simulink model "sf_tictacflow_sim"  (Simulink 6.0)
settings: Solver=ode45  StartTime=0.0  StopTime=inf  RelTol=1e-3
libraries: simulink3 x1
settings Model: CovMetricSettings=dcmtr  Creator=The MathWorks Inc.  LastModifiedBy=batserve  ExtModeTrigMode=oneshot  ExtModeArmWhenConnect=off  ExtModeAutoUpdateStatusClock=off
settings DataIOCC: LimitDataPoints=off  SaveOutput=off  SaveTime=off
settings OptimizationCC: BlockReduction=off  BooleanDataType=off
settings DebuggingCC: CheckExecutionContextPreStartOutputMsg=on  CheckExecutionContextRuntimeOutputMsg=on  SolverPrmCheckMsg=none
settings HardwareCC: TargetUnknown=on

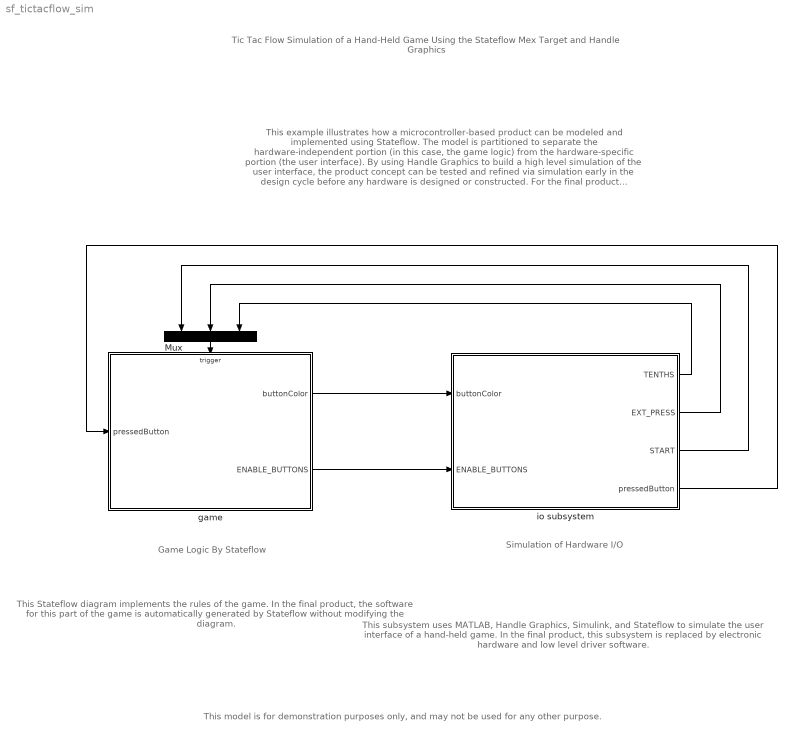
== system sf_tictacflow_sim ==
  note: Tic Tac Flow
      | Simulation of a Hand-Held Game
      | Using the Stateflow Mex Target
      | and Handle Graphics
  note: This model is for demonstration purposes only, and may not be used for any other purpose.
  note: This Stateflow diagram implements
      | the rules of the game.
      |
      | In the final product, the software for this
      | part of the game is automatically generated
      |  by Stateflow without modifying the diagram.
  note: Game Logic By Stateflow
  note: This subsystem uses MATLAB, Handle
      | Graphics, Simulink, and Stateflow
      |  to simulate the user interface of a
      | hand-held game.
      |
      | In the final product, this subsystem is
      | replaced by electronic hardware and
      | low level driver software.
  note: Simulation of Hardware I/O
  note: This example illustrates how a microcontroller-based product can be modeled and implemented using Stateflow.
      |
      | The model is partitioned to separate the hardware-independent portion (in
      | this case, the game logic) from the hardware-specific portion (the user interface).
      | By using Handle Graphics to build a high level simulation of the user interface, the product concept can
      |  be tested and refined via simulation early in the design cycle before any hardware is designed or constructed.
      | For the final product implementation, the hardware-independent portion is implemented automatically
      |  by Stateflow, while the hardware-specific portion is replaced by actual hardware and low-level driver software.
  Mux : Mux  Orientation=down  Inputs=3
  game : Stateflow chart  TreatAsAtomicUnit=on  PropExecContextAcrossSSBoundary=on
  io subsystem : Subsystem  StopFcn=if ishandle(1.000000); delete(1.000000); end;  PropExecContextAcrossSSBoundary=on
  wires:
  io subsystem/4(pressedButton) -> game/1(pressedButton)
  io subsystem/3(START) -> Mux/1
  io subsystem/2(EXT_PRESS) -> Mux/2
  game/2(ENABLE_BUTTONS) -> io subsystem/2(ENABLE_BUTTONS)
  Mux/1 -> game/Trigger
  game/1(buttonColor) -> io subsystem/1(buttonColor)
  io subsystem/1(TENTHS) -> Mux/3

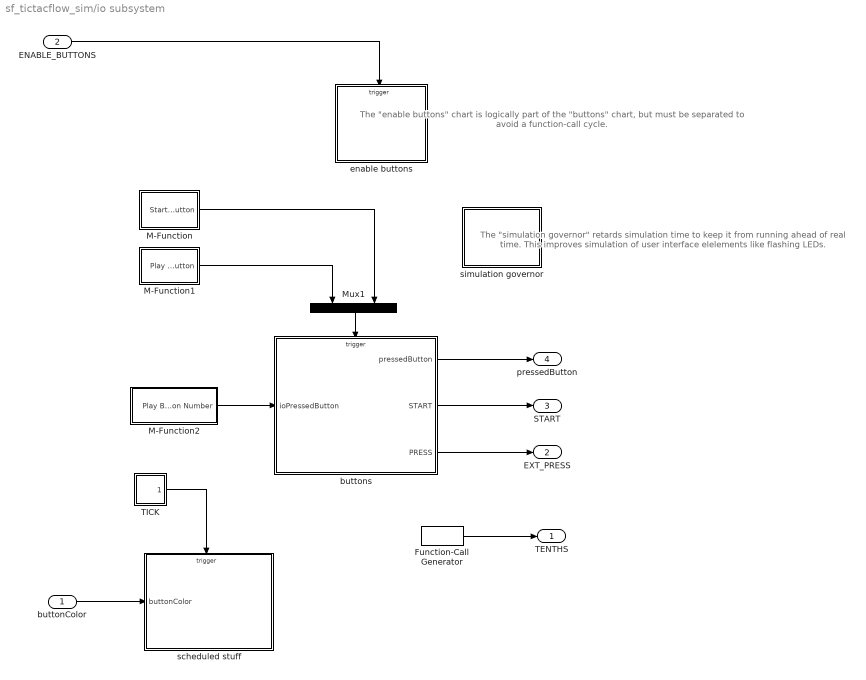
== system sf_tictacflow_sim/io subsystem ==
  note: The "enable buttons" chart is logically part of the
      | "buttons" chart, but must be separated to avoid
      | a function-call cycle.
  note: The "simulation governor" retards simulation time
      | to keep it from running ahead of real time.  This
      | improves simulation of user interface elelements
      | like flashing LEDs.
  buttonColor : Inport  Port=1  LatchInput=off
  ENABLE_BUTTONS : Inport  Port=2  LatchInput=off
  Function-Call Generator : simulink3/Signals & Systems/Function-Call Generator  sample_time=0.1  numberOfIterations=1
  M-Function : Subsystem  PropExecContextAcrossSSBoundary=on
  M-Function1 : Subsystem  PropExecContextAcrossSSBoundary=on
  M-Function2 : Subsystem  PropExecContextAcrossSSBoundary=on
  Mux1 : Mux  Orientation=down  Inputs=2
  TICK : Subsystem  PropExecContextAcrossSSBoundary=on  mask(Pulse Generator){period=1/20, duty=50, amplitude=1, start=0}
      mask prompts: period "Period (secs):"; duty "Duty cycle (% of period):"; start "Start time:"
      mask help: Pulse Generator
      mask Help: Pulse generator which ensures pulse transitions are hit. Provides a vector of pulses when the height is entered as a vector.  Unmask to see how it works.
      mask Display: plot(0,0,100,100,[95,90,90,75,75,60,60,45,45,30,30,15,15,5],[25,25,75,75,25,25,75,75,25,25,75,75,25,25]);
  buttons : Stateflow chart  TreatAsAtomicUnit=on  PropExecContextAcrossSSBoundary=on
  enable buttons : Stateflow chart  TreatAsAtomicUnit=on  PropExecContextAcrossSSBoundary=on
  scheduled stuff : Stateflow chart  TreatAsAtomicUnit=on  PropExecContextAcrossSSBoundary=on
  simulation governor : Subsystem  PropExecContextAcrossSSBoundary=on
  TENTHS : Outport
  EXT_PRESS : Outport  Port=2
  START : Outport  Port=3
  pressedButton : Outport  Port=4
  wires:
  buttons/3(PRESS) -> EXT_PRESS/1
  Mux1/1 -> buttons/Trigger
  buttons/1(pressedButton) -> pressedButton/1
  buttons/2(START) -> START/1
  Function-Call Generator/1 -> TENTHS/1
  M-Function2/1(Play Button Number) -> buttons/1(ioPressedButton)
  buttonColor/1 -> scheduled stuff/1(buttonColor)
  TICK/1(Out1) -> scheduled stuff/Trigger
  M-Function/1(Start Button) -> Mux1/2
  M-Function1/1(Play Button) -> Mux1/1
  ENABLE_BUTTONS/1 -> enable buttons/Trigger

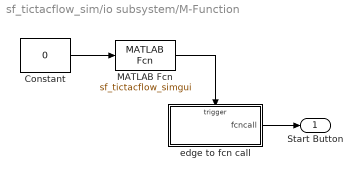
== system sf_tictacflow_sim/io subsystem/M-Function ==
  Constant : Constant  Value=0
  MATLAB Fcn : MATLABFcn  MATLABFcn=sf_tictacflow_simgui
  edge to fcn call : Stateflow chart  TreatAsAtomicUnit=on  PropExecContextAcrossSSBoundary=on
  Start Button : Outport
  wires:
  Constant/1 -> MATLAB Fcn/1
  MATLAB Fcn/1 -> edge to fcn call/Trigger
  edge to fcn call/1(fcncall) -> Start Button/1

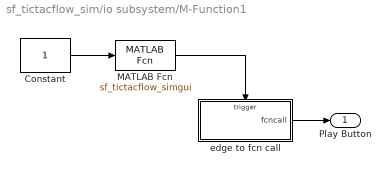
== system sf_tictacflow_sim/io subsystem/M-Function1 ==
  Constant : Constant
  MATLAB Fcn : MATLABFcn  MATLABFcn=sf_tictacflow_simgui
  edge to fcn call : Stateflow chart  TreatAsAtomicUnit=on  PropExecContextAcrossSSBoundary=on
  Play Button : Outport
  wires:
  Constant/1 -> MATLAB Fcn/1
  MATLAB Fcn/1 -> edge to fcn call/Trigger
  edge to fcn call/1(fcncall) -> Play Button/1

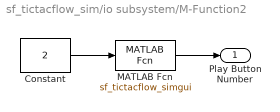
== system sf_tictacflow_sim/io subsystem/M-Function2 ==
  Constant : Constant  Value=2
  MATLAB Fcn : MATLABFcn  MATLABFcn=sf_tictacflow_simgui
  Play Button Number : Outport
  wires:
  MATLAB Fcn/1 -> Play Button Number/1
  Constant/1 -> MATLAB Fcn/1

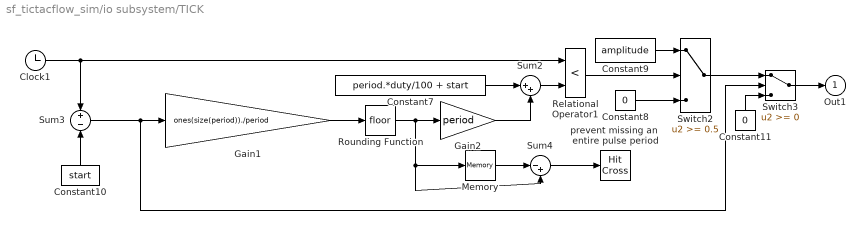
== system sf_tictacflow_sim/io subsystem/TICK ==
  Clock1 : Clock
      settings: Decimation=10
  Constant10 : Constant  Orientation=up  Value=start
  Constant11 : Constant  Orientation=up  Value=0
  Constant7 : Constant  Value=period.*duty/100 + start
  Constant8 : Constant  Value=0
  Constant9 : Constant  Value=amplitude
  Gain1 : Gain  Gain=ones(size(period))./period  SaturateOnIntegerOverflow=on
  Gain2 : Gain  Gain=period  SaturateOnIntegerOverflow=on
  Memory : Memory
  Relational Operator1 : RelationalOperator  Operator=<  InputSameDT=on
  Rounding Function : Rounding
  Sum2 : Sum  Inputs=|++  SaturateOnIntegerOverflow=on  InputSameDT=on
  Sum3 : Sum  Inputs=+-  SaturateOnIntegerOverflow=on  InputSameDT=on
  Sum4 : Sum  Inputs=|-+  SaturateOnIntegerOverflow=on  InputSameDT=on
  Switch2 : Switch  Threshold=0.5  SaturateOnIntegerOverflow=on  InputSameDT=on
  Switch3 : Switch  SaturateOnIntegerOverflow=on  InputSameDT=on
  prevent missing an  entire pulse period : HitCross  HitCrossingOffset=1  ShowOutputPort=off
  Out1 : Outport
  wires:
  Constant10/1 -> Sum3/2
  Sum3/1 -> Gain1/1, Switch3/2
  Clock1/1 -> Relational Operator1/1, Sum3/1
  Sum2/1 -> Relational Operator1/2
  Gain1/1 -> Rounding Function/1
  Constant7/1 -> Sum2/1
  Gain2/1 -> Sum2/2
  Rounding Function/1 -> Sum4/2, Memory/1, Gain2/1
  Switch3/1 -> Out1/1
  Relational Operator1/1 -> Switch2/2
  Constant8/1 -> Switch2/3
  Constant9/1 -> Switch2/1
  Constant11/1 -> Switch3/3
  Switch2/1 -> Switch3/1
  Sum4/1 -> prevent missing an  entire pulse period/1
  Memory/1 -> Sum4/1

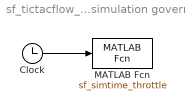
== system sf_tictacflow_sim/io subsystem/simulation governor ==
  Clock : Clock
      settings: Decimation=10
  MATLAB Fcn : MATLABFcn  MATLABFcn=sf_simtime_throttle  OutputDimensions=0
  wires:
  Clock/1 -> MATLAB Fcn/1

== stateflow chart io subsystem/M-Function1/edge to fcn call ==
  (default) -> (junction 3) : { fcncall; }
  events: edge input EITHER_EDGE_EVENT; fcncall output FUNCTION_CALL_EVENT

== stateflow chart io subsystem/M-Function/edge to fcn call ==
  (default) -> (junction 9) : { fcncall; }
  events: edge input EITHER_EDGE_EVENT; fcncall output FUNCTION_CALL_EVENT

== stateflow chart io subsystem/enable buttons ==
  settings: executeAtInitialization=1
  state enable_buttons
    on ENABLE_BUTTONS:
    ml.set(buttonH[0],'Enable','On');
    ml.set(buttonH[1],'Enable','On');
    ml.set(buttonH[2],'Enable','On');
    ml.set(buttonH[3],'Enable','On');
    ml.set(buttonH[4],'Enable','On');
    ml.set(buttonH[5],'Enable','On');
    ml.set(buttonH[6],'Enable','On');
    ml.set(buttonH[7],'Enable','On');
    ml.set(buttonH[8],'Enable','On');
  events: ENABLE_BUTTONS input FUNCTION_CALL_EVENT

== stateflow chart game ==
  settings: executeAtInitialization=1
  state button_7 [parallel]
    state enabled
      buttonColor[thisButton] = DARK;
    state disabled
    state active
      state red
        buttonColor[thisButton] = RED;
        TURN;
      state green
        buttonColor[thisButton] = GREEN;
        TURN;
      (junction 85) -> button_7.active.red
      (junction 85) -> button_7.active.green : [in(turn.green)]
    button_7 -> button_7.disabled : GAME_OVER
    button_7 -> button_7.enabled : START
    (default) -> button_7.enabled
    button_7.active -> button_7.enabled : at(7,TURN)
    button_7.enabled -> (junction 85) : PRESS
  state button_0 [parallel]
    state disabled
    state enabled
      buttonColor[thisButton] = DARK;
    state active
      state red
        buttonColor[thisButton] = RED;
        TURN;
      state green
        buttonColor[thisButton] = GREEN;
        TURN;
      (junction 86) -> button_0.active.red
      (junction 86) -> button_0.active.green : [in(turn.green)]
    button_0 -> button_0.disabled : GAME_OVER
    button_0 -> button_0.enabled : START
    (default) -> button_0.enabled
    button_0.active -> button_0.enabled : at(7,TURN)
    button_0.enabled -> (junction 86) : PRESS
  state button_5 [parallel]
    state disabled
    state enabled
      buttonColor[thisButton] = DARK;
    state active
      state red
        buttonColor[thisButton] = RED;
        TURN;
      state green
        buttonColor[thisButton] = GREEN;
        TURN;
      (junction 87) -> button_5.active.red
      (junction 87) -> button_5.active.green : [in(turn.green)]
    button_5 -> button_5.enabled : START
    button_5 -> button_5.disabled : GAME_OVER
    (default) -> button_5.enabled
    button_5.active -> button_5.enabled : at(7,TURN)
    button_5.enabled -> (junction 87) : PRESS
  state button_2 [parallel]
    state disabled
    state enabled
      buttonColor[thisButton] = DARK;
    state active
      state red
        buttonColor[thisButton] = RED;
        TURN;
      state green
        buttonColor[thisButton] = GREEN;
        TURN;
      (junction 88) -> button_2.active.red
      (junction 88) -> button_2.active.green : [in(turn.green)]
    button_2 -> button_2.disabled : GAME_OVER
    button_2 -> button_2.enabled : START
    (default) -> button_2.enabled
    button_2.active -> button_2.enabled : at(7,TURN)
    button_2.enabled -> (junction 88) : PRESS
  state button_4 [parallel]
    state disabled
    state enabled
      buttonColor[thisButton] = DARK;
    state active
      state red
        buttonColor[thisButton] = RED;
        TURN;
      state green
        buttonColor[thisButton] = GREEN;
        TURN;
      (junction 89) -> button_4.active.red
      (junction 89) -> button_4.active.green : [in(turn.green)]
    button_4 -> button_4.enabled : START
    button_4 -> button_4.disabled : GAME_OVER
    (default) -> button_4.enabled
    button_4.active -> button_4.enabled : at(7,TURN)
    button_4.enabled -> (junction 89) : PRESS
  state button_6 [parallel]
    state disabled
    state enabled
      buttonColor[thisButton] = DARK;
    state active
      state red
        buttonColor[thisButton] = RED;
        TURN;
      state green
        buttonColor[thisButton] = GREEN;
        TURN;
      (junction 90) -> button_6.active.red
      (junction 90) -> button_6.active.green : [in(turn.green)]
    button_6 -> button_6.enabled : START
    button_6 -> button_6.disabled : GAME_OVER
    (default) -> button_6.enabled
    button_6.active -> button_6.enabled : at(7,TURN)
    button_6.enabled -> (junction 90) : PRESS
  state button_3 [parallel]
    state disabled
    state enabled
      buttonColor[thisButton] = DARK;
    state active
      state red
        buttonColor[thisButton] = RED;
        TURN;
      state green
        buttonColor[thisButton] = GREEN;
        TURN;
      (junction 91) -> button_3.active.red
      (junction 91) -> button_3.active.green : [in(turn.green)]
    button_3 -> button_3.enabled : START
    button_3 -> button_3.disabled : GAME_OVER
    (default) -> button_3.enabled
    button_3.active -> button_3.enabled : at(7,TURN)
    button_3.enabled -> (junction 91) : PRESS
  state button_8 [parallel]
    state disabled
    state enabled
      buttonColor[thisButton] = DARK;
    state active
      state red
        buttonColor[thisButton] = RED;
        TURN;
      state green
        buttonColor[thisButton] = GREEN;
        TURN;
      (junction 92) -> button_8.active.red
      (junction 92) -> button_8.active.green : [in(turn.green)]
    button_8 -> button_8.enabled : START
    button_8 -> button_8.disabled : GAME_OVER
    (default) -> button_8.enabled
    button_8.active -> button_8.enabled : at(7,TURN)
    button_8.enabled -> (junction 92) : PRESS
  state button_1 [parallel]
    state disabled
    state enabled
      buttonColor[thisButton] = DARK;
    state active
      state red
        buttonColor[thisButton] = RED;
        TURN;
      state green
        buttonColor[thisButton] = GREEN;
        TURN;
      (junction 93) -> button_1.active.red
      (junction 93) -> button_1.active.green : [in(turn.green)]
    button_1 -> button_1.enabled : START
    button_1 -> button_1.disabled : GAME_OVER
    (default) -> button_1.enabled
    button_1.active -> button_1.enabled : at(7,TURN)
    button_1.enabled -> (junction 93) : PRESS
  state turn [parallel]
    state red
      buttonColor[9] = RED;
      on every(2,TENTHS):
      buttonColor[9] ^= RED;
    state move = choose_move() [function]
      (default) -> (junction 94) : /* try to win on this move */
          | { move = 12 - gameState[1] - gameState[3]; }
      (junction 94) -> (junction 95) : [ make_move_if_available(move) ]
      (junction 94) -> (junction 96) : /* else try to block opponent from winning next move */
          | { move = 12 - gameState[0] - gameState[2]; }
      (junction 96) -> (junction 97) : [ make_move_if_available(move) ]
      (junction 96) -> (junction 98) : /* else make a random  move */
          | { move = seed; }
      (junction 99) -> (junction 98)
      (junction 98) -> (junction 100) : {
          |   /* simple linear congruential
          |      pseudo-random sequence:
          |      x = (5x + 3) mod 16 */
          |   move += move << 2;
          |   move += 3;
          |   move &= 0xf;
          | }
      (junction 101) -> (junction 99)
      (junction 100) -> (junction 101) : [!make_move_if_available(move)]
      (junction 100) -> (junction 102) : { seed = move; }
    state game_over
      GAME_OVER;
      state on
        buttonColor[gameState[0]] = winColor;
        buttonColor[gameState[2]] = winColor;
        buttonColor[gameState[4]] = winColor;
      state off
        buttonColor[gameState[0]] = 0;
        buttonColor[gameState[2]] = 0;
        buttonColor[gameState[4]] = 0;
      (default) -> on : { winColor = buttonColor[gameState[0]]; }
      off -> on : after(1,TENTHS)
      on -> off : after(3,TENTHS)
    state yes = is_a_winner() [function]
      (default) -> (junction 103) : { yes =((gameState[0] + gameState[2] + gameState[4]) == 12); }
    state shift_game_state(magicNumber) [function]
      (default) -> (junction 104) : {
          |   gameState[5] = gameState[4];
          |   gameState[4] = gameState[3];
          |   gameState[3] = gameState[2];
          |   gameState[2] = gameState[1];
          |   gameState[1] = gameState[0];
          |   gameState[0] = magicNumber;
          | }
    state yes = make_move_if_available(move) [function]
      (default) -> (junction 105)
      (junction 105) -> (junction 106) : [ move == 0 && in(button_0.enabled)] { shift_game_state(move); send(PRESS,button_0);}
      (junction 105) -> (junction 107)
      (junction 106) -> (junction 108)
      (junction 107) -> (junction 108) : [ move == 1 && in(button_1.enabled)] { shift_game_state(move); send(PRESS,button_1);}
      (junction 107) -> (junction 109)
      (junction 108) -> (junction 110)
      (junction 109) -> (junction 110) : [ move == 2 && in(button_2.enabled)] { shift_game_state(move); send(PRESS,button_2);}
      (junction 109) -> (junction 111)
      (junction 110) -> (junction 112)
      (junction 111) -> (junction 112) : [ move == 3 && in(button_3.enabled)] { shift_game_state(move); send(PRESS,button_3);}
      (junction 111) -> (junction 113)
      (junction 112) -> (junction 114)
      (junction 113) -> (junction 114) : [ move == 4 && in(button_4.enabled)] { shift_game_state(move); send(PRESS,button_4);}
      (junction 113) -> (junction 115)
      (junction 114) -> (junction 116)
      (junction 115) -> (junction 116) : [ move == 5 && in(button_5.enabled)] { shift_game_state(move); send(PRESS,button_5);}
      (junction 115) -> (junction 117)
      (junction 116) -> (junction 118)
      (junction 117) -> (junction 118) : [ move == 6 && in(button_6.enabled)] { shift_game_state(move); send(PRESS,button_6);}
      (junction 117) -> (junction 119)
      (junction 118) -> (junction 120)
      (junction 119) -> (junction 120) : [ move == 7 && in(button_7.enabled)] { shift_game_state(move); send(PRESS,button_7);}
      (junction 119) -> (junction 121)
      (junction 120) -> (junction 122)
      (junction 121) -> (junction 122) : [ move == 8 && in(button_8.enabled)] { shift_game_state(move); send(PRESS,button_8);}
      (junction 121) -> (junction 124) : { yes = 0; }
      (junction 122) -> (junction 123) : { yes = 1; }
    state green
      buttonColor[9] = GREEN;
      state two_player
        ENABLE_BUTTONS;
        on every(2,TENTHS):
        buttonColor[9] ^= GREEN;
      state sleeping
        on after(SLEEP_TIME,TENTHS):
        choose_move();
      (default) -> (junction 125)
      (junction 125) -> two_player : [TWO_PLAYER]
      (junction 125) -> sleeping
    turn -> (junction 126) : EXT_PRESS
    turn -> (junction 128) : START { ENABLE_BUTTONS; }
    (default) -> (junction 128)
    (junction 126) -> (junction 127) : [make_move_if_available( pressedButton )]
    (junction 126) -> (junction 129) : { ENABLE_BUTTONS; }
    (junction 128) -> turn.red : { gameState = 13; }
    turn.red -> (junction 131) : TURN
    (junction 130) -> turn.red : { ENABLE_BUTTONS; }
    (junction 130) -> game_over : [is_a_winner()]
    (junction 131) -> game_over : [ is_a_winner() ]
    turn.green -> (junction 130) : TURN
    (junction 131) -> turn.green
  data: thisButton constant uint8 =7; thisButton constant uint8; thisButton constant uint8 =5; thisButton constant uint8 =2; thisButton constant uint8 =4; thisButton constant uint8 =6; thisButton constant uint8 =3; thisButton constant uint8 =8; thisButton constant uint8 =1; gameState local uint8 size=9; seed local uint8 =13; move function_output uint8; winColor local uint8; FLASH_RATE constant uint8 =2; yes function_output boolean; sum temporary uint8; count temporary uint8; magicNumber function_input uint8; move function_input uint8; yes function_output boolean; SLEEP_TIME local uint8 =7; pressedButton input uint8; buttonColor output uint8 size=10; DARK constant uint8; GREEN constant uint8 =240; RED constant uint8 =15; TWO_PLAYER constant boolean; YELLOW constant uint8 =255
  events: GAME_OVER local EITHER_EDGE_EVENT; PRESS local EITHER_EDGE_EVENT; TURN local EITHER_EDGE_EVENT; START input FUNCTION_CALL_EVENT; EXT_PRESS input FUNCTION_CALL_EVENT; TENTHS input FUNCTION_CALL_EVENT; ENABLE_BUTTONS output FUNCTION_CALL_EVENT

== stateflow chart io subsystem/buttons ==
  settings: executeAtInitialization=1
  state io
    en:
    figH = ml.sf_tictacflow_simgui('fig');
    ml.set(figH,'Pointer','arrow');
    /* note mapping between magic numbers and button location:
    buttonH[magic] = ml.play_button_magic(figH,location,magic);  */
    buttonH[0] = ml.sf_tictacflow_simgui('play_button',figH,1,0);
    buttonH[1] = ml.sf_tictacflow_simgui('play_button',figH,8,1);
    buttonH[2] = ml.sf_tictacflow_simgui('play_button',figH,3,2);
    buttonH[3] = ml.sf_tictacflow_simgui('play_button',figH,6,3);
    buttonH[4] = ml.sf_tictacflow_simgui('play_button',figH,4,4);
    buttonH[5] = ml.sf_tictacflow_simgui('play_button',figH,2,5);
    buttonH[6] = ml.sf_tictacflow_simgui('play_button',figH,5,6);
    buttonH[7] = ml.sf_tictacflow_simgui('play_button',figH,0,7);
    buttonH[8] = ml.sf_tictacflow_simgui('play_button',figH,7,8);
    startButtonH = ml.sf_tictacflow_simgui('start_button',figH);
    turnSignalH = ml.sf_tictacflow_simgui('turn_signal',figH);
    io -> (junction 291)
    (junction 291) -> (junction 292) : IO_START
        | {
        |    pressedButton = 0;
        |    START;
        | }
    (junction 295) -> (junction 293) : IO_PRESS
        | {
        |   ml.set(buttonH[0],'Enable','Off');
        |   ml.set(buttonH[1],'Enable','Off');
        |   ml.set(buttonH[2],'Enable','Off');
        |   ml.set(buttonH[3],'Enable','Off');
        |   ml.set(buttonH[4],'Enable','Off');
        |   ml.set(buttonH[5],'Enable','Off');
        |   ml.set(buttonH[6],'Enable','Off');
        |   ml.set(buttonH[7],'Enable','Off');
        |   ml.set(buttonH[8],'Enable','Off');
        |   pressedButton = ioPressedButton;
        |   PRESS;
        | }
    (junction 295) -> (junction 294)
    (junction 291) -> (junction 295)
  data: startButtonH local double; ioPressedButton input double; pressedButton output uint8
  events: IO_PRESS input FUNCTION_CALL_EVENT; IO_START input FUNCTION_CALL_EVENT; START output FUNCTION_CALL_EVENT; PRESS output FUNCTION_CALL_EVENT

== stateflow chart io subsystem/scheduled stuff ==
  settings: executeAtInitialization=1
  state stop [parallel]
    stop -> (junction 312)
    (default) -> (junction 312)
    (junction 312) -> (junction 313) : [ !ml.ishandle(figH) ]
        | { ml.set_param('sf_tictacflow_sim','simulationcommand','stop'); }
  state update_LEDs [parallel]
    update_LEDs -> (junction 314)
    (default) -> (junction 314)
    (junction 314) -> (junction 315) : TICK
        | [ml.ishandle(figH)]
        | {
        |   ml.sf_tictacflow_simgui('set_button_color',buttonH[0],buttonColor[0]);
        |   ml.sf_tictacflow_simgui('set_button_color',buttonH[1],buttonColor[1]);
        |   ml.sf_tictacflow_simgui('set_button_color',buttonH[2],buttonColor[2]);
        |   ml.sf_tictacflow_simgui('set_button_color',buttonH[3],buttonColor[3]);
        |   ml.sf_tictacflow_simgui('set_button_color',buttonH[4],buttonColor[4]);
        |   ml.sf_tictacflow_simgui('set_button_color',buttonH[5],buttonColor[5]);
        |   ml.sf_tictacflow_simgui('set_button_color',buttonH[6],buttonColor[6]);
        |   ml.sf_tictacflow_simgui('set_button_color',buttonH[7],buttonColor[7]);
        |   ml.sf_tictacflow_simgui('set_button_color',buttonH[8],buttonColor[8]);
        |   ml.sf_tictacflow_simgui('set_button_color',turnSignalH,buttonColor[9]);
        | }
  data: buttonColor input uint8 size=10
  events: TICK input EITHER_EDGE_EVENT
